simulink model "distillmpcbasic"  (R2022a)
settings: Solver=ode45  StartTime=0.0  StopTime=95  RelTol=1e-3  EnableMultiTasking=on
values from neighbouring files (symbols this model uses):
  F = Kp + Ki/s + Kd*s/(Tf*s+1)    [F_library.m]    (also in MPC_params.m = Gss_disc.A; common_functions.m = pidtune(G,'PID'))
  G = procest(data,'P1D')    [Estimate_G.m]    (also in MPC_params.m = Gss_disc.B; common_functions.m = tf(Gss))
  N = 5    [MPC_params.m]
  Q1 = diag([10000000 10000000])    [MPC_params.m]
  Q2 = diag([0.1 0.1])    [MPC_params.m]
  Ts = 1    [MPC_params.m]    (also in common_functions.m = 0)
  ubounds = [-2 3; -2.5 2.5]    [MPC_params.m]
  x0 = xstar    [MPC_params.m]
undefined symbols (not defined in the file or in its folder): alpha, F0, L0, M, M0B, M0D, Mz, V0, xF0, xstar
settings Model: Creator=maren  LastModifiedBy=Eric
settings SolverCC: AlgebraicLoopSolver=TrustRegion
settings DataIOCC: LimitDataPoints=on  SaveFormat=Array  SignalLoggingSaveFormat=ModelDataLogs  ReturnWorkspaceOutputs=off
settings OptimizationCC: ExpressionDepthLimit=2147483647  InitFltsAndDblsToZero=on  LifeSpan=inf
settings DebuggingCC: SaveWithParameterizedLinksMsg=none  UnderspecifiedInitializationDetection=Classic  MergeDetectMultiDrivingBlocksExec=none  SolverPrmCheckMsg=warning  FcnCallInpInsideContextMsg=warning  UnconnectedInputMsg=warning  UnconnectedOutputMsg=warning  UnconnectedLineMsg=warning  StateNameClashWarn=warning  SFUnexpectedBacktrackingDiag=warning  SFNoUnconditionalDefaultTransitionDiag=warning  SFExecutionAtInitializationDiag=none  SFMachineParentedDataDiag=warning  ArithmeticOperatorsInVariantConditions=warning
settings HardwareCC: ProdBitPerPointer=32  ProdBitPerSizeT=32  ProdBitPerPtrDiffT=32  ProdLargestAtomicFloat=None  ProdIntDivRoundTo=Undefined  ProdEndianess=Unspecified  ProdWordSize=32  ProdHWDeviceType=32-bit Generic
settings ModelReferenceCC: PropagateSignalLabelsOutOfModel=off
settings CodeAppCC: StateflowObjectComments=on
settings GRTTargetCC: TargetFcnLib=ansi_tfl_tmw.mat  TargetLangStandard=C89/C90 (ANSI)  CombineOutputUpdateFcns=off  GRTInterface=on
settings ConfigComp: CovMetricSettings=dw  CovSaveCumulativeToWorkspaceVar=on  CovSaveSingleToWorkspaceVar=on

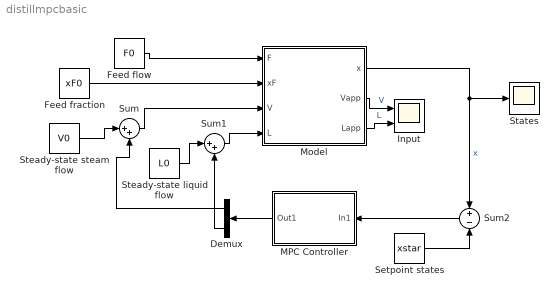
== system distillmpcbasic ==
  Demux : Demux  Outputs=2
      settings: DisplayOption=none
  Feed flow : Constant  Value=F0
  Feed fraction : Constant  Value=xF0
  Input : Scope  NumInputPorts=2
  MPC Controller : Subsystem  mask{F=F, G=G, M=Mz, N=N, Q1=Q1, Q2=Q2, ubounds=ubounds, Ts=Ts, ufname='solvempcproblem'}
      mask prompts: ubounds "Input bounds [u1min u1max;u2min u2max;...]"; ufname "Output function (Ex: 'myfun1')"
      mask Display:
      | port_label('input',1,'x')
      | port_label('output',1,'u')
  Model : Subsystem
  Setpoint states : Constant  Value=xstar
  States : Scope
  Steady-state liquid flow : Constant  Value=L0
  Steady-state steam flow : Constant  Value=V0
  Sum : Sum  Inputs=|++  SaturateOnIntegerOverflow=on
  Sum1 : Sum  Inputs=|++  SaturateOnIntegerOverflow=on
  Sum2 : Sum  Inputs=+-  SaturateOnIntegerOverflow=on
  wires:
  Feed flow/1 -> Model/1(F)
  Feed fraction/1 -> Model/2(xF)
  Steady-state steam flow/1 -> Sum/1
  Sum/1 -> Model/3(V)
  Steady-state liquid flow/1 -> Sum1/1
  Sum1/1 -> Model/4(L)
  Model/2(Vapp) -> Input/1  "V"
  Model/3(Lapp) -> Input/2  "L"
  Setpoint states/1 -> Sum2/2
  Sum2/1 -> MPC Controller/1(In1)
  MPC Controller/1(Out1) -> Demux/1
  Model/1(x) -> Sum2/1, States/1  "x"
  Demux/1 -> Sum/2
  Demux/2 -> Sum1/2

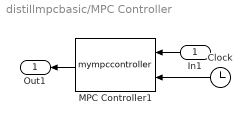
== system distillmpcbasic/MPC Controller ==
  In1 : Inport
  Clock : Clock
  MPC Controller1 : M-S-Function  FunctionName=mympccontroller  Parameters=F,G,M,N,Q1,Q2,ubounds,Ts,ufname  mask{F=F, G=G, M=M, N=N, Q1=Q1, Q2=Q2, ubounds=ubounds, Ts=Ts, ufname=ufname}
      mask prompts: ubounds "ubounds [u1min u1max;u2min u2max;...]"; ufname "Output function (Ex: 'myfun1')"
      mask Display:
      | port_label('input',1,'x')
      | port_label('input',2,'t')
      | port_label('output',1,'u')
  Out1 : Outport
  wires:
  Clock/1 -> MPC Controller1/2
  In1/1 -> MPC Controller1/1
  MPC Controller1/1 -> Out1/1

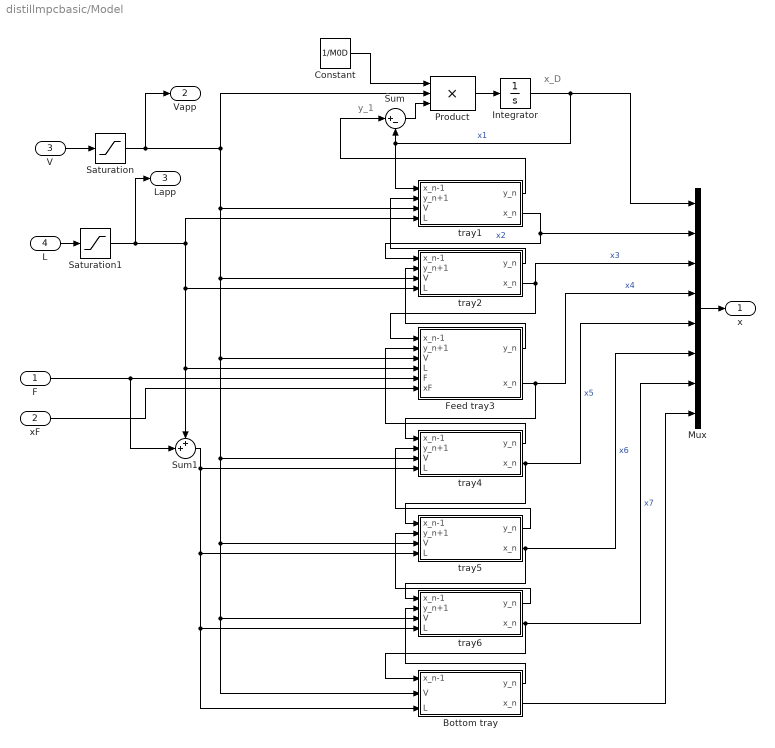
== system distillmpcbasic/Model ==
  note: y_1
  note: x_D
  F : Inport
  xF : Inport  Port=2
  V : Inport  Port=3
  L : Inport  Port=4
  Bottom tray : Subsystem
  Constant : Constant  Value=1/M0D
  Feed tray3 : Subsystem
  Integrator : Integrator  InitialCondition=x0(1)
  Mux : Mux  Inputs=8
  Product : Product  Inputs=3  SaturateOnIntegerOverflow=on  OutDataTypeStr=Inherit: Same as first input
  Saturation : Saturate  UpperLimit=5  LowerLimit=0
  Saturation1 : Saturate  UpperLimit=5  LowerLimit=0
  Sum : Sum  Inputs=|+-  SaturateOnIntegerOverflow=on
  Sum1 : Sum  Inputs=++|  SaturateOnIntegerOverflow=on
  tray1 : Subsystem
  tray2 : Subsystem
  tray4 : Subsystem
  tray5 : Subsystem
  tray6 : Subsystem
  x : Outport
  Vapp : Outport  Port=2
  Lapp : Outport  Port=3
  wires:
  L/1 -> Saturation1/1
  V/1 -> Saturation/1
  Mux/1 -> x/1
  Bottom tray/2(x_n) -> Mux/8
  tray6/2(x_n) -> Bottom tray/1(x_n-1), Mux/7  "x7"
  Bottom tray/1(y_n) -> tray6/2(y_n+1)
  Sum1/1 -> Bottom tray/3(L), tray6/4(L), tray5/4(L), tray4/4(L)
  tray5/2(x_n) -> tray6/1(x_n-1), Mux/6  "x6"
  tray6/1(y_n) -> tray5/2(y_n+1)
  tray4/2(x_n) -> tray5/1(x_n-1), Mux/5  "x5"
  tray5/1(y_n) -> tray4/2(y_n+1)
  Feed tray3/2(x_n) -> Mux/4, tray4/1(x_n-1)  "x4"
  tray4/1(y_n) -> Feed tray3/2(y_n+1)
  xF/1 -> Feed tray3/6(xF)
  F/1 -> Sum1/2, Feed tray3/5(F)
  tray2/2(x_n) -> Mux/3, Feed tray3/1(x_n-1)  "x3"
  Feed tray3/1(y_n) -> tray2/2(y_n+1)
  tray1/2(x_n) -> Mux/2, tray2/1(x_n-1)  "x2"
  tray2/1(y_n) -> tray1/2(y_n+1)
  tray1/1(y_n) -> Sum/1
  Saturation1/1 -> Lapp/1, tray1/4(L), Sum1/1, Feed tray3/4(L), tray2/4(L)
  Saturation/1 -> Vapp/1, Bottom tray/2(V), tray6/3(V), tray5/3(V), tray4/3(V), Feed tray3/3(V), tray2/3(V), tray1/3(V), Product/2
  Sum/1 -> Product/3
  Constant/1 -> Product/1
  Product/1 -> Integrator/1
  Integrator/1 -> Mux/1, tray1/1(x_n-1), Sum/2  "x1"

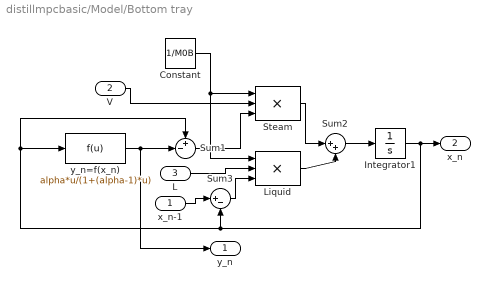
== system distillmpcbasic/Model/Bottom tray ==
  x_n-1 : Inport
  V : Inport  Port=2
  L : Inport  Port=3
  Constant : Constant  Value=1/M0B
  Integrator1 : Integrator  InitialCondition=x0(8)
  Liquid : Product  Inputs=3  SaturateOnIntegerOverflow=on  OutDataTypeStr=Inherit: Same as first input
  Steam : Product  Inputs=3  SaturateOnIntegerOverflow=on  OutDataTypeStr=Inherit: Same as first input
  Sum1 : Sum  Inputs=+-|  SaturateOnIntegerOverflow=on
  Sum2 : Sum  Inputs=|++  SaturateOnIntegerOverflow=on
  Sum3 : Sum  Inputs=|+-  SaturateOnIntegerOverflow=on
  y_n=f(x_n) : Fcn  Expr=alpha*u/(1+(alpha-1)*u)
  y_n : Outport
  x_n : Outport  Port=2
  wires:
  Sum1/1 -> Steam/3
  Constant/1 -> Steam/1, Liquid/1
  Integrator1/1 -> x_n/1, Sum1/1, y_n=f(x_n)/1, Sum3/2
  y_n=f(x_n)/1 -> y_n/1, Sum1/2
  V/1 -> Steam/2
  Liquid/1 -> Sum2/2
  Steam/1 -> Sum2/1
  Sum2/1 -> Integrator1/1
  L/1 -> Liquid/2
  x_n-1/1 -> Sum3/1
  Sum3/1 -> Liquid/3

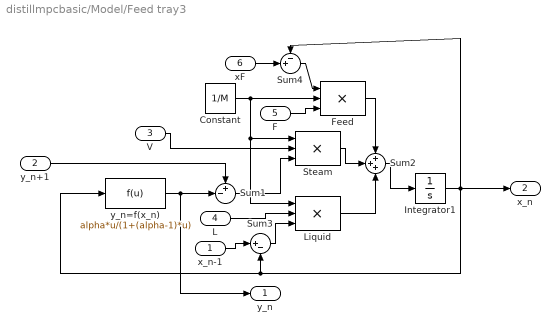
== system distillmpcbasic/Model/Feed tray3 ==
  x_n-1 : Inport
  y_n+1 : Inport  Port=2
  V : Inport  Port=3
  L : Inport  Port=4
  F : Inport  Port=5
  xF : Inport  Port=6
  Constant : Constant  Value=1/M
  Feed : Product  Inputs=3  SaturateOnIntegerOverflow=on  OutDataTypeStr=Inherit: Same as first input
  Integrator1 : Integrator  InitialCondition=x0(4)
  Liquid : Product  Inputs=3  SaturateOnIntegerOverflow=on  OutDataTypeStr=Inherit: Same as first input
  Steam : Product  Inputs=3  SaturateOnIntegerOverflow=on  OutDataTypeStr=Inherit: Same as first input
  Sum1 : Sum  Inputs=+-|  SaturateOnIntegerOverflow=on
  Sum2 : Sum  Inputs=+++  SaturateOnIntegerOverflow=on
  Sum3 : Sum  Inputs=|+-  SaturateOnIntegerOverflow=on
  Sum4 : Sum  Inputs=-+|  SaturateOnIntegerOverflow=on
  y_n=f(x_n) : Fcn  Expr=alpha*u/(1+(alpha-1)*u)
  y_n : Outport
  x_n : Outport  Port=2
  wires:
  Feed/1 -> Sum2/1
  Sum4/1 -> Feed/1
  F/1 -> Feed/3
  xF/1 -> Sum4/2
  Steam/1 -> Sum2/2
  Liquid/1 -> Sum2/3
  Sum1/1 -> Steam/3
  Constant/1 -> Steam/1, Liquid/1, Feed/2
  Integrator1/1 -> Sum4/1, x_n/1, y_n=f(x_n)/1, Sum3/2
  y_n=f(x_n)/1 -> y_n/1, Sum1/2
  y_n+1/1 -> Sum1/1
  V/1 -> Steam/2
  Sum2/1 -> Integrator1/1
  L/1 -> Liquid/2
  x_n-1/1 -> Sum3/1
  Sum3/1 -> Liquid/3

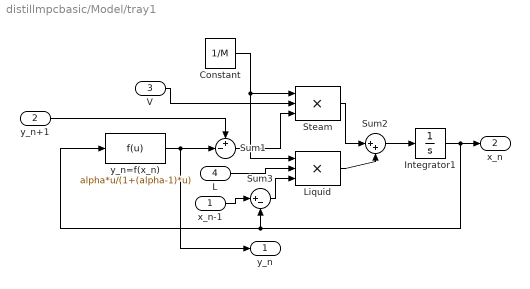
== system distillmpcbasic/Model/tray1 ==
  x_n-1 : Inport
  y_n+1 : Inport  Port=2
  V : Inport  Port=3
  L : Inport  Port=4
  Constant : Constant  Value=1/M
  Integrator1 : Integrator  InitialCondition=x0(2)
  Liquid : Product  Inputs=3  SaturateOnIntegerOverflow=on  OutDataTypeStr=Inherit: Same as first input
  Steam : Product  Inputs=3  SaturateOnIntegerOverflow=on  OutDataTypeStr=Inherit: Same as first input
  Sum1 : Sum  Inputs=+-|  SaturateOnIntegerOverflow=on
  Sum2 : Sum  Inputs=|++  SaturateOnIntegerOverflow=on
  Sum3 : Sum  Inputs=|+-  SaturateOnIntegerOverflow=on
  y_n=f(x_n) : Fcn  Expr=alpha*u/(1+(alpha-1)*u)
  y_n : Outport
  x_n : Outport  Port=2
  wires:
  Sum1/1 -> Steam/3
  Constant/1 -> Steam/1, Liquid/1
  Integrator1/1 -> x_n/1, y_n=f(x_n)/1, Sum3/2
  y_n=f(x_n)/1 -> y_n/1, Sum1/2
  y_n+1/1 -> Sum1/1
  V/1 -> Steam/2
  Liquid/1 -> Sum2/2
  Steam/1 -> Sum2/1
  Sum2/1 -> Integrator1/1
  L/1 -> Liquid/2
  x_n-1/1 -> Sum3/1
  Sum3/1 -> Liquid/3

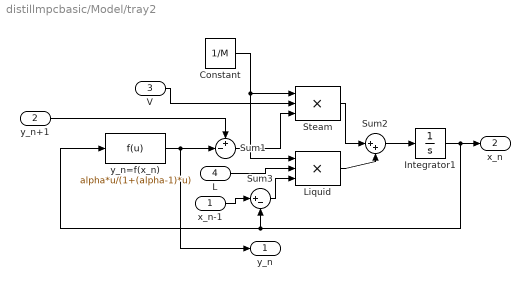
== system distillmpcbasic/Model/tray2 ==
  x_n-1 : Inport
  y_n+1 : Inport  Port=2
  V : Inport  Port=3
  L : Inport  Port=4
  Constant : Constant  Value=1/M
  Integrator1 : Integrator  InitialCondition=x0(3)
  Liquid : Product  Inputs=3  SaturateOnIntegerOverflow=on  OutDataTypeStr=Inherit: Same as first input
  Steam : Product  Inputs=3  SaturateOnIntegerOverflow=on  OutDataTypeStr=Inherit: Same as first input
  Sum1 : Sum  Inputs=+-|  SaturateOnIntegerOverflow=on
  Sum2 : Sum  Inputs=|++  SaturateOnIntegerOverflow=on
  Sum3 : Sum  Inputs=|+-  SaturateOnIntegerOverflow=on
  y_n=f(x_n) : Fcn  Expr=alpha*u/(1+(alpha-1)*u)
  y_n : Outport
  x_n : Outport  Port=2
  wires:
  Sum3/1 -> Liquid/3
  x_n-1/1 -> Sum3/1
  L/1 -> Liquid/2
  Sum2/1 -> Integrator1/1
  Steam/1 -> Sum2/1
  Liquid/1 -> Sum2/2
  V/1 -> Steam/2
  y_n+1/1 -> Sum1/1
  y_n=f(x_n)/1 -> Sum1/2, y_n/1
  Integrator1/1 -> Sum3/2, y_n=f(x_n)/1, x_n/1
  Constant/1 -> Liquid/1, Steam/1
  Sum1/1 -> Steam/3

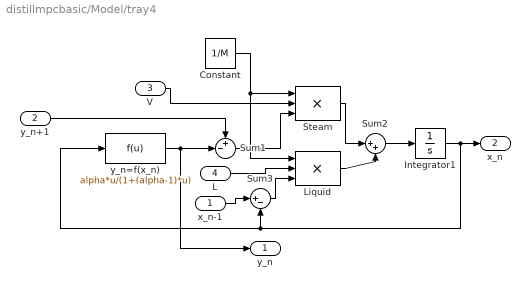
== system distillmpcbasic/Model/tray4 ==
  x_n-1 : Inport
  y_n+1 : Inport  Port=2
  V : Inport  Port=3
  L : Inport  Port=4
  Constant : Constant  Value=1/M
  Integrator1 : Integrator  InitialCondition=x0(5)
  Liquid : Product  Inputs=3  SaturateOnIntegerOverflow=on  OutDataTypeStr=Inherit: Same as first input
  Steam : Product  Inputs=3  SaturateOnIntegerOverflow=on  OutDataTypeStr=Inherit: Same as first input
  Sum1 : Sum  Inputs=+-|  SaturateOnIntegerOverflow=on
  Sum2 : Sum  Inputs=|++  SaturateOnIntegerOverflow=on
  Sum3 : Sum  Inputs=|+-  SaturateOnIntegerOverflow=on
  y_n=f(x_n) : Fcn  Expr=alpha*u/(1+(alpha-1)*u)
  y_n : Outport
  x_n : Outport  Port=2
  wires:
  Sum3/1 -> Liquid/3
  x_n-1/1 -> Sum3/1
  L/1 -> Liquid/2
  Sum2/1 -> Integrator1/1
  Steam/1 -> Sum2/1
  Liquid/1 -> Sum2/2
  V/1 -> Steam/2
  y_n+1/1 -> Sum1/1
  y_n=f(x_n)/1 -> Sum1/2, y_n/1
  Integrator1/1 -> Sum3/2, y_n=f(x_n)/1, x_n/1
  Constant/1 -> Liquid/1, Steam/1
  Sum1/1 -> Steam/3

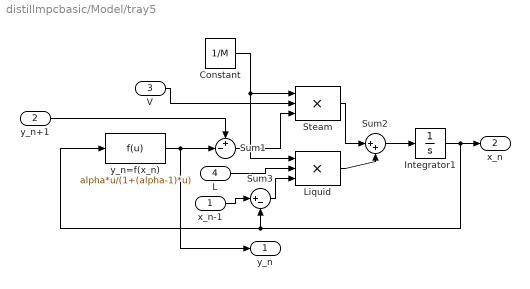
== system distillmpcbasic/Model/tray5 ==
  x_n-1 : Inport
  y_n+1 : Inport  Port=2
  V : Inport  Port=3
  L : Inport  Port=4
  Constant : Constant  Value=1/M
  Integrator1 : Integrator  InitialCondition=x0(6)
  Liquid : Product  Inputs=3  SaturateOnIntegerOverflow=on  OutDataTypeStr=Inherit: Same as first input
  Steam : Product  Inputs=3  SaturateOnIntegerOverflow=on  OutDataTypeStr=Inherit: Same as first input
  Sum1 : Sum  Inputs=+-|  SaturateOnIntegerOverflow=on
  Sum2 : Sum  Inputs=|++  SaturateOnIntegerOverflow=on
  Sum3 : Sum  Inputs=|+-  SaturateOnIntegerOverflow=on
  y_n=f(x_n) : Fcn  Expr=alpha*u/(1+(alpha-1)*u)
  y_n : Outport
  x_n : Outport  Port=2
  wires:
  Sum1/1 -> Steam/3
  Constant/1 -> Steam/1, Liquid/1
  Integrator1/1 -> x_n/1, y_n=f(x_n)/1, Sum3/2
  y_n=f(x_n)/1 -> y_n/1, Sum1/2
  y_n+1/1 -> Sum1/1
  V/1 -> Steam/2
  Liquid/1 -> Sum2/2
  Steam/1 -> Sum2/1
  Sum2/1 -> Integrator1/1
  L/1 -> Liquid/2
  x_n-1/1 -> Sum3/1
  Sum3/1 -> Liquid/3

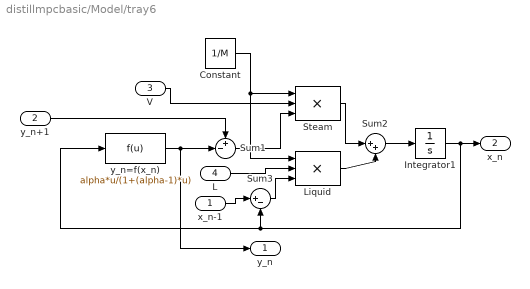
== system distillmpcbasic/Model/tray6 ==
  x_n-1 : Inport
  y_n+1 : Inport  Port=2
  V : Inport  Port=3
  L : Inport  Port=4
  Constant : Constant  Value=1/M
  Integrator1 : Integrator  InitialCondition=x0(7)
  Liquid : Product  Inputs=3  SaturateOnIntegerOverflow=on  OutDataTypeStr=Inherit: Same as first input
  Steam : Product  Inputs=3  SaturateOnIntegerOverflow=on  OutDataTypeStr=Inherit: Same as first input
  Sum1 : Sum  Inputs=+-|  SaturateOnIntegerOverflow=on
  Sum2 : Sum  Inputs=|++  SaturateOnIntegerOverflow=on
  Sum3 : Sum  Inputs=|+-  SaturateOnIntegerOverflow=on
  y_n=f(x_n) : Fcn  Expr=alpha*u/(1+(alpha-1)*u)
  y_n : Outport
  x_n : Outport  Port=2
  wires:
  Sum3/1 -> Liquid/3
  x_n-1/1 -> Sum3/1
  L/1 -> Liquid/2
  Sum2/1 -> Integrator1/1
  Steam/1 -> Sum2/1
  Liquid/1 -> Sum2/2
  V/1 -> Steam/2
  y_n+1/1 -> Sum1/1
  y_n=f(x_n)/1 -> Sum1/2, y_n/1
  Integrator1/1 -> Sum3/2, y_n=f(x_n)/1, x_n/1
  Constant/1 -> Liquid/1, Steam/1
  Sum1/1 -> Steam/3
